simulink model "S2File_JD2016MMSS"  (R2017a)
settings: Solver=VariableStepAuto  StartTime=0.0  StopTime=96  RelTol=1e-3  EnableMultiTasking=on
settings Model: Creator=mathiasfoo  LastModifiedBy=ac8227
settings OptimizationCC: LifeSpan=inf
settings DebuggingCC: SFUnexpectedBacktrackingDiag=warning  SFNoUnconditionalDefaultTransitionDiag=warning  SFExecutionAtInitializationDiag=none
settings GRTTargetCC: TargetLangStandard=C89/C90 (ANSI)  GeneratePreprocessorConditionals=Disable all
settings ConfigComp: CovMetricSettings=dw  CovHtmlReporting=on  CovSaveCumulativeToWorkspaceVar=on  CovSaveSingleToWorkspaceVar=on  CovExternalEMLEnable=off

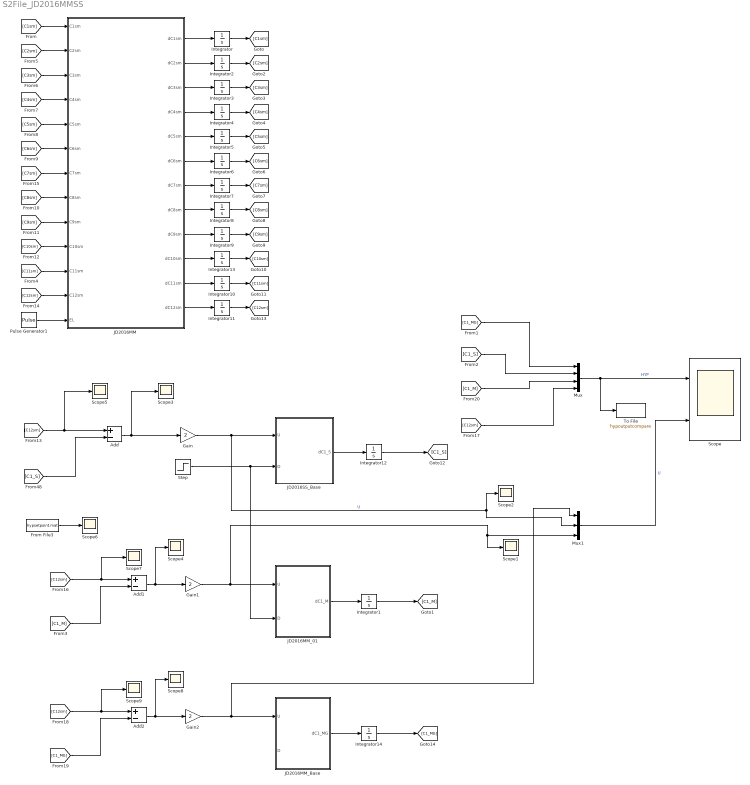
== system S2File_JD2016MMSS ==
  Add : Sum  Inputs=+-
  Add1 : Sum  Inputs=+-
  Add2 : Sum  Inputs=+-
  From File3 : FromFile  FileName=hypsetpoint.mat  SampleTime=0
  Gain : Gain  Gain=2
  Gain1 : Gain  Gain=2
  Gain2 : Gain  Gain=2
  Integrator{,1,12,14} (4 alike) : Integrator  InitialCondition=1.3627
  Integrator10 : Integrator  InitialCondition=0.0938
  Integrator11 : Integrator  InitialCondition=6.2713
  Integrator13 : Integrator  InitialCondition=0.5547
  Integrator2 : Integrator  InitialCondition=2.2647
  Integrator3 : Integrator  InitialCondition=0.9724
  Integrator4 : Integrator  InitialCondition=0.9495
  Integrator5 : Integrator  InitialCondition=0.1906
  Integrator6 : Integrator  InitialCondition=0.4318
  Integrator7 : Integrator  InitialCondition=0.0332
  Integrator8 : Integrator  InitialCondition=0.0189
  Integrator9 : Integrator  InitialCondition=0.3578
  JD2016MM : MATLAB Function  TreatAsAtomicUnit=on
  JD2016MM_01 : MATLAB Function  TreatAsAtomicUnit=on
  JD2016MM_Base : MATLAB Function  TreatAsAtomicUnit=on
  JD2016SS_Base : MATLAB Function  TreatAsAtomicUnit=on
  Mux : Mux
  Mux1 : Mux  Inputs=3
  Pulse Generator1 : DiscretePulseGenerator  PulseType=Time based  Period=24  PulseWidth=50
  Scope : Scope  NumInputPorts=2
  Scope{1..9} (9 alike) : Scope
  Step : Step  Time=50  After=-0.01  SampleTime=0
  To File : ToFile  Filename=hypoutputcompare  MatrixName=yhyp
  wires:
  Integrator12/1 -> [C1_S]
  Step/1 -> JD2016MM_01/2(D), JD2016SS_Base/2(D)
  Add/1 -> Gain/1, Scope3/1
  JD2016SS_Base/1(dC1_S) -> Integrator12/1
  Mux/1 -> Scope/1, To File/1  "HYP"
  JD2016MM_01/1(dC1_M) -> Integrator1/1
  Integrator1/1 -> [C1_M]
  [C12sm] -> Scope7/1, Add1/1
  Add1/1 -> Gain1/1, Scope4/1
  Gain1/1 -> Scope1/1, Mux1/3, JD2016MM_01/1(U)
  Gain/1 -> JD2016SS_Base/1(U), Mux1/2, Scope2/1  "U"
  Mux1/1 -> Scope/2  "U"
  [C1_MG] -> Mux/1
  [C1_S] -> Mux/2
  From File3/1 -> Scope6/1
  [C12sm] -> Scope5/1, Add/1
  [C3sm] -> JD2016MM/3(C3sm)
  [C4sm] -> JD2016MM/4(C4sm)
  Pulse Generator1/1 -> JD2016MM/13(EL)
  Integrator4/1 -> [C4sm]
  Integrator2/1 -> [C2sm]
  JD2016MM/2(dC2sm) -> Integrator2/1
  [C2sm] -> JD2016MM/2(C2sm)
  Integrator5/1 -> [C5sm]
  [C6sm] -> JD2016MM/6(C6sm)
  Integrator13/1 -> [C10sm]
  [C11sm] -> JD2016MM/11(C11sm)
  JD2016MM/10(dC10sm) -> Integrator13/1
  JD2016MM/3(dC3sm) -> Integrator3/1
  [C5sm] -> JD2016MM/5(C5sm)
  Integrator7/1 -> [C7sm]
  Integrator9/1 -> [C9sm]
  Integrator6/1 -> [C6sm]
  [C1sm] -> JD2016MM/1(C1sm)
  JD2016MM/12(dC12sm) -> Integrator11/1
  Integrator10/1 -> [C11sm]
  Integrator/1 -> [C1sm]
  Integrator3/1 -> [C3sm]
  JD2016MM/1(dC1sm) -> Integrator/1
  JD2016MM/6(dC6sm) -> Integrator6/1
  JD2016MM/9(dC9sm) -> Integrator9/1
  JD2016MM/11(dC11sm) -> Integrator10/1
  [C9sm] -> JD2016MM/9(C9sm)
  [C12sm] -> JD2016MM/12(C12sm)
  [C7sm] -> JD2016MM/7(C7sm)
  [C8sm] -> JD2016MM/8(C8sm)
  JD2016MM/4(dC4sm) -> Integrator4/1
  JD2016MM/8(dC8sm) -> Integrator8/1
  Integrator11/1 -> [C12sm]
  [C10sm] -> JD2016MM/10(C10sm)
  JD2016MM/7(dC7sm) -> Integrator7/1
  Integrator8/1 -> [C8sm]
  JD2016MM/5(dC5sm) -> Integrator5/1
  [C1_S] -> Add/2
  [C1_M] -> Add1/2
  Integrator14/1 -> [C1_MG]
  JD2016MM_Base/1(dC1_MG) -> Integrator14/1
  [C1_MG] -> Add2/2
  [C12sm] -> Scope9/1, Add2/1
  Add2/1 -> Gain2/1, Scope8/1
  Gain2/1 -> Mux1/1, JD2016MM_Base/1(U)
  [C1_M] -> Mux/3
  [C12sm] -> Mux/4

== matlab function S2File_JD2016MMSS/JD2016SS_Base ==
  data: dC1_S output; U input; D input
function dC1_S = fcn(U,D)

%% For HYP phenotype
% % Base Value (MSE = 0.0313)
% prmLHY = [0.72294,-1.2502,-0.042071,0.75237,-0.97172];
% prpLHY = [0.80635,0.74888,0.74688];
% prmP97 = [0.026394,0.12407,-2.3687,-0.10561,0.35392,1.5597];
% prpP97 = [1.0733,0.29692,-0.050611];
% prmP51 = [0.38365,-0.71673,0.17357,1.013];
% prpP51 = [0.55202,0.41674,-0.27927];
% prmEL = [0.010977,-1.8819,-1.3932,-0.017199,0.48139];
% prpEL = [1.0696,1.3282,0.91055];
% prpP = [0.34819,0.36754,-0.64076];
% prmPIF = [0.036342,-0.28081,0.19706];
% prpPIF = [0.30969,0.18321,-2.0456];
% prpHYP = [0.17399,1.1843];

% % Range ~50/100
% prmLHY = [0.72294,-1.2502,-0.042071,0.75237,-0.97172];
% prpLHY = [0.80635,0.74888,0.74688];
% prmP97 = [0.026394,0.12407,-2.3687,-0.10561,0.35392,1.5597];
% prpP97 = [1.0733,0.29692,-0.050611];
% prmP51 = [0.38365,-0.71673,0.17357,1.013];
% prpP51 = [0.55202,0.41674,-0.27927];
% prmEL = [0.010977,-1.8819,-1.3932,-0.017199,0.48139];
% prpEL = [1.0696,1.3282,0.91055];
% prpP = [0.34819,0.36754,-0.64076];
% prmPIF = [0.036342,-0.28081,0.19706];
% prpPIF = [0.30969,0.18321,-2.0456];
% prpHYP = [0.15802,1.1583];              % Converges to ~1
% % prpHYP = [3200223873895.316,50]; % (Fix at 50 in ODE, poor fit)

% % Range ~5/10
% prmLHY = [0.72294,-1.2502,-0.042071,0.75237,-0.97172];
% prpLHY = [0.80635,0.74888,0.74688];
% prmP97 = [0.026394,0.12407,-2.3687,-0.10561,0.35392,1.5597];
% prpP97 = [1.0733,0.29692,-0.050611];
% prmP51 = [0.38365,-0.71673,0.17357,1.013];
% prpP51 = [0.55202,0.41674,-0.27927];
% prmEL = [0.010977,-1.8819,-1.3932,-0.017199,0.48139];
% prpEL = [1.0696,1.3282,0.91055];
% prpP = [0.34819,0.36754,-0.64076];
% prmPIF = [0.036342,-0.28081,0.19706];
% prpPIF = [0.30969,0.18321,-2.0456];
% prpHYP = [0.13709,1.0517];       % Converges to ~1
% % prpHYP = [4.7245,5]; % (Fix at 5 in ODE, poor fit)
% 
% 
% % Range ~0.5/0.1
% prmLHY = [0.72294,-1.2502,-0.042071,0.75237,-0.97172];
% prpLHY = [0.80635,0.74888,0.74688];
% prmP97 = [0.026394,0.12407,-2.3687,-0.10561,0.35392,1.5597];
% prpP97 = [1.0733,0.29692,-0.050611];
% prmP51 = [0.38365,-0.71673,0.17357,1.013];
% prpP51 = [0.55202,0.41674,-0.27927];
% prmEL = [0.010977,-1.8819,-1.3932,-0.017199,0.48139];
% prpEL = [1.0696,1.3282,0.91055];
% prpP = [0.34819,0.36754,-0.64076];
% prmPIF = [0.036342,-0.28081,0.19706];
% prpPIF = [0.30969,0.18321,-2.0456];
% prpHYP = [0.11376,0.91571];      % Converges to ~1
% % prpHYP = [0.059094,0.5]; % (Fix at 0.5 in ODE, decent fit)
% 
% % Range ~0.05/0.01
% prmLHY = [0.72294,-1.2502,-0.042071,0.75237,-0.97172];
% prpLHY = [0.80635,0.74888,0.74688];
% prmP97 = [0.026394,0.12407,-2.3687,-0.10561,0.35392,1.5597];
% prpP97 = [1.0733,0.29692,-0.050611];
% prmP51 = [0.38365,-0.71673,0.17357,1.013];
% prpP51 = [0.55202,0.41674,-0.27927];
% prmEL = [0.010977,-1.8819,-1.3932,-0.017199,0.48139];
% prpEL = [1.0696,1.3282,0.91055];
% prpP = [0.34819,0.36754,-0.64076];
% prmPIF = [0.036342,-0.28081,0.19706];
% prpPIF = [0.30969,0.18321,-2.0456];
% prpHYP = [0.11378,0.91588];         % Converges to ~1
% % prpHYP = [0.025615,0.05]; % (Fix at 0.05 in ODE, straight line fit)
% 
% Range ~0.005/0.001
prmLHY = [0.72294,-1.2502,-0.042071,0.75237,-0.97172];
prpLHY = [0.80635,0.74888,0.74688];
prmP97 = [0.026394,0.12407,-2.3687,-0.10561,0.35392,1.5597];
prpP97 = [1.0733,0.29692,-0.050611];
prmP51 = [0.38365,-0.71673,0.17357,1.013];
prpP51 = [0.55202,0.41674,-0.27927];
prmEL = [0.010977,-1.8819,-1.3932,-0.017199,0.48139];
prpEL = [1.0696,1.3282,0.91055];
prpP = [0.34819,0.36754,-0.64076];
prmPIF = [0.036342,-0.28081,0.19706];
prpPIF = [0.30969,0.18321,-2.0456];
prpHYP = [0.11375,0.91564];        % Converges to ~1
% % prpHYP = [0.023389,0.005]; % (Fix at 0.005 in ODE, straight line fit)

theta = [prmLHY prpLHY prmP97 prpP97 prmP51 prpP51 prmEL prpEL prpP prmPIF prpPIF prpHYP];

% % LHY mRNA
% dC1_S = real(theta(1)*C4_S^(theta(2))*C6_S^(theta(3)) - theta(4)*C1_S + theta(5)*C9_S*EL);
% 
% % LHY protein
% dC2_S = real(theta(6)*C1_S - theta(7)*C2_S + theta(8)*EL*C1_S);
% 
% % P97 mRNA
% dC3_S = real(theta(9)*C2_S^(theta(10))*C6_S^(theta(11))*C8_S^(theta(12)) - theta(13)*C3_S + theta(14)*C9_S*EL);
% 
% % P97 protein
% dC4_S = real(theta(15)*C3_S - theta(16)*C4_S + theta(17)*EL*C4_S);
% 
% % P51 mRNA
% dC5_S = real(theta(18)*C2_S^(theta(19))*C6_S^(theta(20)) - theta(21)*C5_S);
%  
% % P51 protein
% dC6_S = real(theta(22)*C5_S - theta(23)*C6_S + theta(24)*EL*C6_S);
% 
% % EL mRNA
% dC7_S = real(theta(25)*C2_S^(theta(26))*C6_S^(theta(27))*C8_S^(theta(28))*EL - theta(29)*C7_S);
% 
% % EL protein
% dC8_S = real(theta(30)*C7_S - theta(31)*C8_S + theta(32)*EL*C8_S);
% 
% % Protein P
% dC9_S = real(theta(33)*(1-EL) - theta(34)*C9_S*(1-EL) + theta(35)*EL*C9_S);
% 
% % PIF mRNA
% dC10_S = real(theta(36)*C8_S^(theta(37)) - theta(38)*C10_S);
% 
% % PIF protein
% dC11_S = real(theta(39)*C10_S - theta(40)*C11_S + theta(41)*EL*C11_S);

% HYP protein
% dC1_S = real(theta(42)*C11_S^theta(43));

dC1_S = real((theta(42)*(real(U^theta(43))) + 0*(D)));

== matlab function S2File_JD2016MMSS/JD2016MM_01 ==
  data: dC1_M output; U input; D input
function dC1_M = fcn(U,D)

% % Base Value
% prmLHY = [1.5593,3.1251,8.5131,0.52816,0.57095,0.27846];
% prpLHY = [1.4223,1.6312,1.2323];
% prmP97 = [6.6492,1.0127,1.1825,0.27924,4.3706,5.9883,0.21494];
% prpP97 = [1.4474,0.98029,0.4934];
% prmP51 = [1.029,1.6903,0.3192,0.6966];
% prpP51 = [0.71371,0.50082,0.79076];
% prmEL = [1.8696,3.412,0.98472,0.44702,0.71066];
% prpEL = [4.4692,4.2413,2.5113];
% prpP = [0.30156,0.31029,1.032];
% prmPIF = [0.11429,3.5332,0.16961];
% prpPIF = [2.0499,2.7462,16.1476];
% prpHYP = [0.0085946,0.1217,0.45243];

% % Range ~50
% prmLHY = [2.3435,3.0753,9.1718,0.69925,0.46285,0.22089];
% prpLHY = [1.6073,1.6019,1.585];
% prmP97 = [3.823,3.9184,0.45925,133.7882,3.7811,0.35601,0.70223];
% prpP97 = [1.0835,0.45186,0.3232];
% prmP51 = [1.1266,2.2945,0.45965,0.62393];
% prpP51 = [0.58279,0.44605,0.62256];
% prmEL = [2.2276,3.5244,1.3601,0.0098821,0.78759];
% prpEL = [4.0757,3.706,2.1514];
% prpP = [0.51362,0.58512,1.781];
% prmPIF = [0.097235,3.1304,0.15472];
% prpPIF = [2.2853,2.5682,13.6595];
% prpHYP = [0.0064573,1.1479,1.7883];

% % Range ~5
% prmLHY = [1.3416,3.6527,7.1504,0.55057,0.52728,0.24401];
% prpLHY = [1.5542,1.9979,1.5031];
% prmP97 = [7.374,1.5806,1.8515,5.4146,3.4513,3.033,0.27101];
% prpP97 = [1.4459,0.95351,0.46207];
% prmP51 = [0.97723,1.8055,0.36245,0.59841];
% prpP51 = [0.56828,0.43465,0.72829];
% prmEL = [1.9677,3.2416,1.2408,0.46046,0.71489];
% prpEL = [4.7441,3.6836,2.5884];
% prpP = [0.29656,0.32051,1.0503];
% prmPIF = [0.11092,3.2451,0.16639];
% prpPIF = [2.2008,2.5697,17.1694];
% prpHYP = [0.010777,0.1263,0.66981];

% % Range ~0.05
% prmLHY = [2.7098,3.4495,10.8631,0.6676,0.47202,0.26469];
% prpLHY = [1.594,1.7178,1.4976];
% prmP97 = [3.3176,1.2539,1.1743,0.065826,3.7187,3.0973,0.36593];
% prpP97 = [1.2095,0.51557,0.33537];
% prmP51 = [1.0577,1.8419,0.25522,0.72493];
% prpP51 = [0.67839,0.48974,0.71074];
% prmEL = [2.608,3.6233,1.357,0.32897,0.77942];
% prpEL = [2.1579,3.2993,1.1068];
% prpP = [0.34968,0.38151,1.2377];
% prmPIF = [0.10463,2.1977,0.18435];
% prpPIF = [2.6251,2.989,19.0262];
% prpHYP = [0.010044,0.12346,0.63408];

% % Range ~0.005
% prmLHY = [1.6297,3.0362,7.7067,0.53067,0.37992,0.28016];
% prpLHY = [1.5987,1.8819,1.7831];
% prmP97 = [6.2698,1.0317,1.5606,0.0056269,3.8126,3.5392,0.26747];
% prpP97 = [1.1902,0.93133,0.42344];
% prmP51 = [1.1629,1.8773,0.40229,0.68638];
% prpP51 = [0.67085,0.47213,0.73036];
% prmEL = [2.4313,2.6744,1.2014,0.48639,0.74646];
% prpEL = [4.3937,3.6608,2.4211];
% prpP = [0.30285,0.31329,1.0213];
% prmPIF = [0.114,3.786,0.16502];
% prpPIF = [2.2741,2.5594,18.1271];
% prpHYP = [0.010621,0.12189,0.55233];

% % Range ~0.0005
% prmLHY = [2.6568,3.2435,13.28,0.60431,0.48325,0.19928];
% prpLHY = [1.4361,1.6692,1.4153];
% prmP97 = [4.2153,0.61749,2.1085,0.00053005,3.3815e-4,4.4862,0.33641];
% prpP97 = [0.93011,0.57615,0.27266];
% prmP51 = [1.1641,1.9336,0.23137,0.79026];
% prpP51 = [0.52447,0.401,0.5448];
% prmEL = [2.8458,4.2769,1.5747,0.14401,0.80917];
% prpEL = [5.2188,4.5847,2.7603];
% prpP = [0.50575,0.57446,1.4607];
% prmPIF = [0.095406,2.9158,0.15432];
% prpPIF = [1.8453,2.0869,11.5701];
% prpHYP = [0.0094957,0.074354,0.36446];

%% For HYP phenotype
% % Base value
% prmLHY = [4.6,3,39.0625,0.6944,0.53,0.21];
% prpLHY = [0.76,0.42,0.68];
% prmP97 = [5,1.3,1.5,0.0576,18.9036,11.1111,0.35];
% prpP97 = [1,0.5,0.3];
% prmP51 = [1,4.7259,0.25,0.56];
% prpP51 = [0.64,0.48,0.78];
% prmEL = [1.5,7.716,0.277,0.277,0.57];
% prpEL = [1,1.2,0.38];
% prpP = [0.3,0.3,1];
% prmPIF = [0.1,22.6757,0.14];
% prpPIF = [0.62,0.52,4];
% prpHYP = [0.01,0.12,0.3136];

% % Range ~100
% prmLHY = [4.6,3,39.0625,0.6944,0.53,0.21];
% prpLHY = [0.76,0.42,0.68];
% prmP97 = [5,1.3,1.5,0.0576,18.9036,11.1111,0.35];
% prpP97 = [1,0.5,0.3];
% prmP51 = [1,4.7259,0.25,0.56];
% prpP51 = [0.64,0.48,0.78];
% prmEL = [1.5,7.716,0.277,0.277,0.57];
% prpEL = [1,1.2,0.38];
% prpP = [0.3,0.3,1];
% prmPIF = [0.1,22.6757,0.14];
% prpPIF = [0.62,0.52,4];
% prpHYP = [0.015156,14.4749,100.3136];

% % Range ~10
% prmLHY = [4.6,3,39.0625,0.6944,0.53,0.21];
% prpLHY = [0.76,0.42,0.68];
% prmP97 = [5,1.3,1.5,0.0576,18.9036,11.1111,0.35];
% prpP97 = [1,0.5,0.3];
% prmP51 = [1,4.7259,0.25,0.56];
% prpP51 = [0.64,0.48,0.78];
% prmEL = [1.5,7.716,0.277,0.277,0.57];
% prpEL = [1,1.2,0.38];
% prpP = [0.3,0.3,1];
% prmPIF = [0.1,22.6757,0.14];
% prpPIF = [0.62,0.52,4];
% prpHYP = [0.010513,2.336,10.0454];

% % Range ~0.1
% prmLHY = [4.6,3,39.0625,0.6944,0.53,0.21];
% prpLHY = [0.76,0.42,0.68];
% prmP97 = [5,1.3,1.5,0.0576,18.9036,11.1111,0.35];
% prpP97 = [1,0.5,0.3];
% prmP51 = [1,4.7259,0.25,0.56];
% prpP51 = [0.64,0.48,0.78];
% prmEL = [1.5,7.716,0.277,0.277,0.57];
% prpEL = [1,1.2,0.38];
% prpP = [0.3,0.3,1];
% prmPIF = [0.1,22.6757,0.14];
% prpPIF = [0.62,0.52,4];
% prpHYP = [0.0049959,0.088027,0.12667];

% % Range ~0.01
% prmLHY = [4.6,3,39.0625,0.6944,0.53,0.21];
% prpLHY = [0.76,0.42,0.68];
% prmP97 = [5,1.3,1.5,0.0576,18.9036,11.1111,0.35];
% prpP97 = [1,0.5,0.3];
% prmP51 = [1,4.7259,0.25,0.56];
% prpP51 = [0.64,0.48,0.78];
% prmEL = [1.5,7.716,0.277,0.277,0.57];
% prpEL = [1,1.2,0.38];
% prpP = [0.3,0.3,1];
% prmPIF = [0.1,22.6757,0.14];
% prpPIF = [0.62,0.52,4];
% prpHYP = [0.0048173,0.037503,0.01667];

% Range ~0.001
prmLHY = [4.6,3,39.0625,0.6944,0.53,0.21];
prpLHY = [0.76,0.42,0.68];
prmP97 = [5,1.3,1.5,0.0576,18.9036,11.1111,0.35];
prpP97 = [1,0.5,0.3];
prmP51 = [1,4.7259,0.25,0.56];
prpP51 = [0.64,0.48,0.78];
prmEL = [1.5,7.716,0.277,0.277,0.57];
prpEL = [1,1.2,0.38];
prpP = [0.3,0.3,1];
prmPIF = [0.1,22.6757,0.14];
prpPIF = [0.62,0.52,4];
prpHYP = [0.0003814,0.03772,0.0083637];


theta = [prmLHY prpLHY prmP97 prpP97 prmP51 prpP51 prmEL prpEL prpP prmPIF prpPIF prpHYP];

% % LHY mRNA
% dC1_S = (theta(1) + theta(2)*EL*C9_S)/(1 + theta(3)*C4_S^2 + theta(4)*C6_S^2) - (theta(5)*EL + theta(6)*(1-EL))*C1_S;
% 
% % LHY protein
% dC2_S = (theta(7) + theta(8)*EL)*C1_S - theta(9)*C2_S;
% 
% % P97 mRNA
% dC3_S = (theta(10)*EL*C9_S + theta(11) + (theta(12)*(0*U + 1*C2_S^2))/(theta(13)^2 + (0*U + 1*C2_S^2)))*(1/(1 + theta(14)^2*C6_S^2 + theta(15)^2*C8_S^2)) ...
%     - theta(16)*C3_S;
% 
% % P97 protein
% dC4_S = theta(17)*C3_S - theta(18)*(1-EL)*C4_S - theta(19)*EL*C4_S;
% 
% % P51 mRNA
% dC5_S = theta(20)/(1 + theta(21)^2*C2_S^2 + theta(22)^2*C6_S^2) - theta(23)*C5_S;
% 
% % P51 protein
% dC6_S = theta(24)*C5_S - theta(25)*(1-EL)*C6_S - theta(26)*EL*C6_S;
% 
% % EL mRNA
% dC7_S = theta(27)*EL/(1 + theta(28)^2*C2_S^2 + theta(29)^2*C6_S^2 + theta(30)^2*C8_S^2) - theta(31)*C7_S;
% 
% % EL protein
% dC8_S = theta(32)*C7_S - theta(33)*(1-EL)*C8_S - theta(34)*EL*C8_S;
% 
% % Protein P
% dC9_S = theta(35)*(1-EL) - theta(36)*C9_S*(1-EL) - theta(37)*EL*C9_S;
% 
% % PIF mRNA
% dC10_S = theta(38)/(1 + theta(39)^2*C8_S^2) - theta(40)*C10_S;
% 
% % PIF protein
% dC11_S = theta(41)*C10_S - theta(42)*(1-EL)*C11_S - theta(43)*EL*C11_S;
% 
% % HYP protein
% dC12_S = theta(44) + (theta(45)*(1*U + 0*C11_S^2))/(theta(46)^2 + (1*U + 0*C11_S^2)) + D;

dC1_M = theta(44) + (theta(45)*(1*U))/(theta(46)^2 + (1*U)) + 0*D;

== matlab function S2File_JD2016MMSS/JD2016MM_Base ==
  data: dC1_MG output; U input; D input
function dC1_MG = fcn(U,D)

% % Base Value
% prmLHY = [1.5593,3.1251,8.5131,0.52816,0.57095,0.27846];
% prpLHY = [1.4223,1.6312,1.2323];
% prmP97 = [6.6492,1.0127,1.1825,0.27924,4.3706,5.9883,0.21494];
% prpP97 = [1.4474,0.98029,0.4934];
% prmP51 = [1.029,1.6903,0.3192,0.6966];
% prpP51 = [0.71371,0.50082,0.79076];
% prmEL = [1.8696,3.412,0.98472,0.44702,0.71066];
% prpEL = [4.4692,4.2413,2.5113];
% prpP = [0.30156,0.31029,1.032];
% prmPIF = [0.11429,3.5332,0.16961];
% prpPIF = [2.0499,2.7462,16.1476];
% prpHYP = [0.0085946,0.1217,0.45243];

% % Range ~50
% prmLHY = [2.3435,3.0753,9.1718,0.69925,0.46285,0.22089];
% prpLHY = [1.6073,1.6019,1.585];
% prmP97 = [3.823,3.9184,0.45925,133.7882,3.7811,0.35601,0.70223];
% prpP97 = [1.0835,0.45186,0.3232];
% prmP51 = [1.1266,2.2945,0.45965,0.62393];
% prpP51 = [0.58279,0.44605,0.62256];
% prmEL = [2.2276,3.5244,1.3601,0.0098821,0.78759];
% prpEL = [4.0757,3.706,2.1514];
% prpP = [0.51362,0.58512,1.781];
% prmPIF = [0.097235,3.1304,0.15472];
% prpPIF = [2.2853,2.5682,13.6595];
% prpHYP = [0.0064573,1.1479,1.7883];

% % Range ~5
% prmLHY = [1.3416,3.6527,7.1504,0.55057,0.52728,0.24401];
% prpLHY = [1.5542,1.9979,1.5031];
% prmP97 = [7.374,1.5806,1.8515,5.4146,3.4513,3.033,0.27101];
% prpP97 = [1.4459,0.95351,0.46207];
% prmP51 = [0.97723,1.8055,0.36245,0.59841];
% prpP51 = [0.56828,0.43465,0.72829];
% prmEL = [1.9677,3.2416,1.2408,0.46046,0.71489];
% prpEL = [4.7441,3.6836,2.5884];
% prpP = [0.29656,0.32051,1.0503];
% prmPIF = [0.11092,3.2451,0.16639];
% prpPIF = [2.2008,2.5697,17.1694];
% prpHYP = [0.010777,0.1263,0.66981];

% % Range ~0.05
% prmLHY = [2.7098,3.4495,10.8631,0.6676,0.47202,0.26469];
% prpLHY = [1.594,1.7178,1.4976];
% prmP97 = [3.3176,1.2539,1.1743,0.065826,3.7187,3.0973,0.36593];
% prpP97 = [1.2095,0.51557,0.33537];
% prmP51 = [1.0577,1.8419,0.25522,0.72493];
% prpP51 = [0.67839,0.48974,0.71074];
% prmEL = [2.608,3.6233,1.357,0.32897,0.77942];
% prpEL = [2.1579,3.2993,1.1068];
% prpP = [0.34968,0.38151,1.2377];
% prmPIF = [0.10463,2.1977,0.18435];
% prpPIF = [2.6251,2.989,19.0262];
% prpHYP = [0.010044,0.12346,0.63408];

% % Range ~0.005
% prmLHY = [1.6297,3.0362,7.7067,0.53067,0.37992,0.28016];
% prpLHY = [1.5987,1.8819,1.7831];
% prmP97 = [6.2698,1.0317,1.5606,0.0056269,3.8126,3.5392,0.26747];
% prpP97 = [1.1902,0.93133,0.42344];
% prmP51 = [1.1629,1.8773,0.40229,0.68638];
% prpP51 = [0.67085,0.47213,0.73036];
% prmEL = [2.4313,2.6744,1.2014,0.48639,0.74646];
% prpEL = [4.3937,3.6608,2.4211];
% prpP = [0.30285,0.31329,1.0213];
% prmPIF = [0.114,3.786,0.16502];
% prpPIF = [2.2741,2.5594,18.1271];
% prpHYP = [0.010621,0.12189,0.55233];

% % Range ~0.0005
% prmLHY = [2.6568,3.2435,13.28,0.60431,0.48325,0.19928];
% prpLHY = [1.4361,1.6692,1.4153];
% prmP97 = [4.2153,0.61749,2.1085,0.00053005,3.3815e-4,4.4862,0.33641];
% prpP97 = [0.93011,0.57615,0.27266];
% prmP51 = [1.1641,1.9336,0.23137,0.79026];
% prpP51 = [0.52447,0.401,0.5448];
% prmEL = [2.8458,4.2769,1.5747,0.14401,0.80917];
% prpEL = [5.2188,4.5847,2.7603];
% prpP = [0.50575,0.57446,1.4607];
% prmPIF = [0.095406,2.9158,0.15432];
% prpPIF = [1.8453,2.0869,11.5701];
% prpHYP = [0.0094957,0.074354,0.36446];

%% For HYP phenotype
% Base value
prmLHY = [4.6,3,39.0625,0.6944,0.53,0.21];
prpLHY = [0.76,0.42,0.68];
prmP97 = [5,1.3,1.5,0.0576,18.9036,11.1111,0.35];
prpP97 = [1,0.5,0.3];
prmP51 = [1,4.7259,0.25,0.56];
prpP51 = [0.64,0.48,0.78];
prmEL = [1.5,7.716,0.277,0.277,0.57];
prpEL = [1,1.2,0.38];
prpP = [0.3,0.3,1];
prmPIF = [0.1,22.6757,0.14];
prpPIF = [0.62,0.52,4];
prpHYP = [0.01,0.12,0.3136];

% % Range ~100
% prmLHY = [4.6,3,39.0625,0.6944,0.53,0.21];
% prpLHY = [0.76,0.42,0.68];
% prmP97 = [5,1.3,1.5,0.0576,18.9036,11.1111,0.35];
% prpP97 = [1,0.5,0.3];
% prmP51 = [1,4.7259,0.25,0.56];
% prpP51 = [0.64,0.48,0.78];
% prmEL = [1.5,7.716,0.277,0.277,0.57];
% prpEL = [1,1.2,0.38];
% prpP = [0.3,0.3,1];
% prmPIF = [0.1,22.6757,0.14];
% prpPIF = [0.62,0.52,4];
% prpHYP = [0.015156,14.4749,100.3136];

% % Range ~10
% prmLHY = [4.6,3,39.0625,0.6944,0.53,0.21];
% prpLHY = [0.76,0.42,0.68];
% prmP97 = [5,1.3,1.5,0.0576,18.9036,11.1111,0.35];
% prpP97 = [1,0.5,0.3];
% prmP51 = [1,4.7259,0.25,0.56];
% prpP51 = [0.64,0.48,0.78];
% prmEL = [1.5,7.716,0.277,0.277,0.57];
% prpEL = [1,1.2,0.38];
% prpP = [0.3,0.3,1];
% prmPIF = [0.1,22.6757,0.14];
% prpPIF = [0.62,0.52,4];
% prpHYP = [0.010513,2.336,10.0454];

% % Range ~0.1
% prmLHY = [4.6,3,39.0625,0.6944,0.53,0.21];
% prpLHY = [0.76,0.42,0.68];
% prmP97 = [5,1.3,1.5,0.0576,18.9036,11.1111,0.35];
% prpP97 = [1,0.5,0.3];
% prmP51 = [1,4.7259,0.25,0.56];
% prpP51 = [0.64,0.48,0.78];
% prmEL = [1.5,7.716,0.277,0.277,0.57];
% prpEL = [1,1.2,0.38];
% prpP = [0.3,0.3,1];
% prmPIF = [0.1,22.6757,0.14];
% prpPIF = [0.62,0.52,4];
% prpHYP = [0.0049959,0.088027,0.12667];

% % Range ~0.01
% prmLHY = [4.6,3,39.0625,0.6944,0.53,0.21];
% prpLHY = [0.76,0.42,0.68];
% prmP97 = [5,1.3,1.5,0.0576,18.9036,11.1111,0.35];
% prpP97 = [1,0.5,0.3];
% prmP51 = [1,4.7259,0.25,0.56];
% prpP51 = [0.64,0.48,0.78];
% prmEL = [1.5,7.716,0.277,0.277,0.57];
% prpEL = [1,1.2,0.38];
% prpP = [0.3,0.3,1];
% prmPIF = [0.1,22.6757,0.14];
% prpPIF = [0.62,0.52,4];
% prpHYP = [0.0048173,0.037503,0.01667];

% % Range ~0.001
% prmLHY = [4.6,3,39.0625,0.6944,0.53,0.21];
% prpLHY = [0.76,0.42,0.68];
% prmP97 = [5,1.3,1.5,0.0576,18.9036,11.1111,0.35];
% prpP97 = [1,0.5,0.3];
% prmP51 = [1,4.7259,0.25,0.56];
% prpP51 = [0.64,0.48,0.78];
% prmEL = [1.5,7.716,0.277,0.277,0.57];
% prpEL = [1,1.2,0.38];
% prpP = [0.3,0.3,1];
% prmPIF = [0.1,22.6757,0.14];
% prpPIF = [0.62,0.52,4];
% prpHYP = [0.0003814,0.03772,0.0083637];


theta = [prmLHY prpLHY prmP97 prpP97 prmP51 prpP51 prmEL prpEL prpP prmPIF prpPIF prpHYP];

% % LHY mRNA
% dC1_S = (theta(1) + theta(2)*EL*C9_S)/(1 + theta(3)*C4_S^2 + theta(4)*C6_S^2) - (theta(5)*EL + theta(6)*(1-EL))*C1_S;
% 
% % LHY protein
% dC2_S = (theta(7) + theta(8)*EL)*C1_S - theta(9)*C2_S;
% 
% % P97 mRNA
% dC3_S = (theta(10)*EL*C9_S + theta(11) + (theta(12)*(0*U + 1*C2_S^2))/(theta(13)^2 + (0*U + 1*C2_S^2)))*(1/(1 + theta(14)^2*C6_S^2 + theta(15)^2*C8_S^2)) ...
%     - theta(16)*C3_S;
% 
% % P97 protein
% dC4_S = theta(17)*C3_S - theta(18)*(1-EL)*C4_S - theta(19)*EL*C4_S;
% 
% % P51 mRNA
% dC5_S = theta(20)/(1 + theta(21)^2*C2_S^2 + theta(22)^2*C6_S^2) - theta(23)*C5_S;
% 
% % P51 protein
% dC6_S = theta(24)*C5_S - theta(25)*(1-EL)*C6_S - theta(26)*EL*C6_S;
% 
% % EL mRNA
% dC7_S = theta(27)*EL/(1 + theta(28)^2*C2_S^2 + theta(29)^2*C6_S^2 + theta(30)^2*C8_S^2) - theta(31)*C7_S;
% 
% % EL protein
% dC8_S = theta(32)*C7_S - theta(33)*(1-EL)*C8_S - theta(34)*EL*C8_S;
% 
% % Protein P
% dC9_S = theta(35)*(1-EL) - theta(36)*C9_S*(1-EL) - theta(37)*EL*C9_S;
% 
% % PIF mRNA
% dC10_S = theta(38)/(1 + theta(39)^2*C8_S^2) - theta(40)*C10_S;
% 
% % PIF protein
% dC11_S = theta(41)*C10_S - theta(42)*(1-EL)*C11_S - theta(43)*EL*C11_S;
% 
% % HYP protein
% dC12_S = theta(44) + (theta(45)*(1*U + 0*C11_S^2))/(theta(46)^2 + (1*U + 0*C11_S^2)) + D;

dC1_MG = theta(44) + (theta(45)*(1*U))/(theta(46)^2 + (1*U)) + 0*D;

== matlab function S2File_JD2016MMSS/JD2016MM ==
  data: C1sm input; dC1sm output; C2sm input; C3sm input; C4sm input; C5sm input; C6sm input; C7sm input; C8sm input; C9sm input; C10sm input; C11sm input; C12sm input; EL input; dC2sm output; dC3sm output; dC4sm output; dC5sm output; dC6sm output; dC7sm output; dC8sm output; dC9sm output; dC10sm output; dC11sm output; dC12sm output
function [dC1sm,dC2sm,dC3sm,dC4sm,dC5sm,dC6sm,dC7sm,dC8sm,dC9sm,dC10sm,dC11sm,dC12sm] ...
    = fcn(C1sm,C2sm,C3sm,C4sm,C5sm,C6sm,C7sm,C8sm,C9sm,C10sm,C11sm,C12sm,EL)

% Base value
prmLHY = [4.6,3,39.0625,0.6944,0.53,0.21];
prpLHY = [0.76,0.42,0.68];
prmP97 = [5,1.3,1.5,sqrt(0.0576),sqrt(18.9036),sqrt(11.1111),0.35];
prpP97 = [1,0.5,0.3];
prmP51 = [1,sqrt(4.7259),sqrt(0.25),0.56];
prpP51 = [0.64,0.48,0.78];
prmEL = [1.5,sqrt(7.716),sqrt(0.277),sqrt(0.277),0.57];
prpEL = [1,1.2,0.38];
prpP = [0.3,0.3,1];
prmPIF = [0.1,sqrt(22.6757),0.14];
prpPIF = [0.62,0.52,4];
prpHYP = [0.01,(0.12),0.3136];

% % Base value
% prmLHY = [4.6,3,39.0625,0.6944,0.53,0.21];
% prpLHY = [0.76,0.42,0.68];
% prmP97 = [5,1.3,1.5,0.0576,18.9036,11.1111,0.35];
% prpP97 = [1,0.5,0.3];
% prmP51 = [1,4.7259,0.25,0.56];
% prpP51 = [0.64,0.48,0.78];
% prmEL = [1.5,7.716,0.277,0.277,0.57];
% prpEL = [1,1.2,0.38];
% prpP = [0.3,0.3,1];
% prmPIF = [0.1,22.6757,0.14];
% prpPIF = [0.62,0.52,4];
% prpHYP = [0.01,0.12,0.3136];

% % Range ~100
% prmLHY = [4.6,3,39.0625,0.6944,0.53,0.21];
% prpLHY = [0.76,0.42,0.68];
% prmP97 = [5,1.3,1.5,0.0576,18.9036,11.1111,0.35];
% prpP97 = [1,0.5,0.3];
% prmP51 = [1,4.7259,0.25,0.56];
% prpP51 = [0.64,0.48,0.78];
% prmEL = [1.5,7.716,0.277,0.277,0.57];
% prpEL = [1,1.2,0.38];
% prpP = [0.3,0.3,1];
% prmPIF = [0.1,22.6757,0.14];
% prpPIF = [0.62,0.52,4];
% prpHYP = [0.015156,14.4749,100.3136];

% % Range ~10
% prmLHY = [4.6,3,39.0625,0.6944,0.53,0.21];
% prpLHY = [0.76,0.42,0.68];
% prmP97 = [5,1.3,1.5,0.0576,18.9036,11.1111,0.35];
% prpP97 = [1,0.5,0.3];
% prmP51 = [1,4.7259,0.25,0.56];
% prpP51 = [0.64,0.48,0.78];
% prmEL = [1.5,7.716,0.277,0.277,0.57];
% prpEL = [1,1.2,0.38];
% prpP = [0.3,0.3,1];
% prmPIF = [0.1,22.6757,0.14];
% prpPIF = [0.62,0.52,4];
% prpHYP = [0.010513,2.336,10.0454];

% % Range ~0.1
% prmLHY = [4.6,3,39.0625,0.6944,0.53,0.21];
% prpLHY = [0.76,0.42,0.68];
% prmP97 = [5,1.3,1.5,0.0576,18.9036,11.1111,0.35];
% prpP97 = [1,0.5,0.3];
% prmP51 = [1,4.7259,0.25,0.56];
% prpP51 = [0.64,0.48,0.78];
% prmEL = [1.5,7.716,0.277,0.277,0.57];
% prpEL = [1,1.2,0.38];
% prpP = [0.3,0.3,1];
% prmPIF = [0.1,22.6757,0.14];
% prpPIF = [0.62,0.52,4];
% prpHYP = [0.0049959,0.088027,0.12667];

% % Range ~0.01
% prmLHY = [4.6,3,39.0625,0.6944,0.53,0.21];
% prpLHY = [0.76,0.42,0.68];
% prmP97 = [5,1.3,1.5,0.0576,18.9036,11.1111,0.35];
% prpP97 = [1,0.5,0.3];
% prmP51 = [1,4.7259,0.25,0.56];
% prpP51 = [0.64,0.48,0.78];
% prmEL = [1.5,7.716,0.277,0.277,0.57];
% prpEL = [1,1.2,0.38];
% prpP = [0.3,0.3,1];
% prmPIF = [0.1,22.6757,0.14];
% prpPIF = [0.62,0.52,4];
% prpHYP = [0.0048173,0.037503,0.01667];

% % Range ~0.001
% prmLHY = [4.6,3,39.0625,0.6944,0.53,0.21];
% prpLHY = [0.76,0.42,0.68];
% prmP97 = [5,1.3,1.5,0.0576,18.9036,11.1111,0.35];
% prpP97 = [1,0.5,0.3];
% prmP51 = [1,4.7259,0.25,0.56];
% prpP51 = [0.64,0.48,0.78];
% prmEL = [1.5,7.716,0.277,0.277,0.57];
% prpEL = [1,1.2,0.38];
% prpP = [0.3,0.3,1];
% prmPIF = [0.1,22.6757,0.14];
% prpPIF = [0.62,0.52,4];
% prpHYP = [0.0003814,0.03772,0.0083637];


theta = [prmLHY prpLHY prmP97 prpP97 prmP51 prpP51 prmEL prpEL prpP prmPIF prpPIF prpHYP];

% LHY mRNA
dC1sm = (theta(1) + theta(2)*EL*C9sm)/(1 + theta(3)*C4sm^2 + theta(4)*C6sm^2) - (theta(5)*EL + theta(6)*(1-EL))*C1sm;

% LHY protein
dC2sm = (theta(7) + theta(8)*EL)*C1sm - theta(9)*C2sm;

% P97 mRNA
dC3sm = (theta(10)*EL*C9sm + theta(11) + (theta(12)*(1*C2sm^2))/(theta(13)^2 + (1*C2sm^2)))*(1/(1 + theta(14)^2*C6sm^2 + theta(15)^2*C8sm^2)) ...
    - theta(16)*C3sm;

% P97 protein
dC4sm = theta(17)*C3sm - theta(18)*(1-EL)*C4sm - theta(19)*EL*C4sm;

% P51 mRNA
dC5sm = theta(20)/(1 + theta(21)^2*C2sm^2 + theta(22)^2*C6sm^2) - theta(23)*C5sm;

% P51 protein
dC6sm = theta(24)*C5sm - theta(25)*(1-EL)*C6sm - theta(26)*EL*C6sm;

% EL mRNA
dC7sm = theta(27)*EL/(1 + theta(28)^2*C2sm^2 + theta(29)^2*C6sm^2 + theta(30)^2*C8sm^2) - theta(31)*C7sm;

% EL protein
dC8sm = theta(32)*C7sm - theta(33)*(1-EL)*C8sm - theta(34)*EL*C8sm;

% Protein P
dC9sm = theta(35)*(1-EL) - theta(36)*C9sm*(1-EL) - theta(37)*EL*C9sm;

% PIF mRNA
dC10sm = theta(38)/(1 + theta(39)^2*C8sm^2) - theta(40)*C10sm;

% PIF protein
dC11sm = theta(41)*C10sm - theta(42)*(1-EL)*C11sm - theta(43)*EL*C11sm;

% HYP protein
dC12sm = theta(44) + (theta(45)*(C11sm^2))/(theta(46)^2 + (C11sm^2));
